simulink model "gaussian"  (R2017a)
settings: Solver=FixedStepDiscrete  StartTime=0.0  StopTime=10.0  RelTol=1e-3
undefined symbols (not defined in the file): gray, none, videoinput
libraries: imaqlib x1, visionfilter x1, visiontransforms x1, visiongeotforms x1, dspmtrx3 x1
settings Model: SimulationMode=accelerator  Creator=eruffaldi  LastModifiedBy=eruffaldi

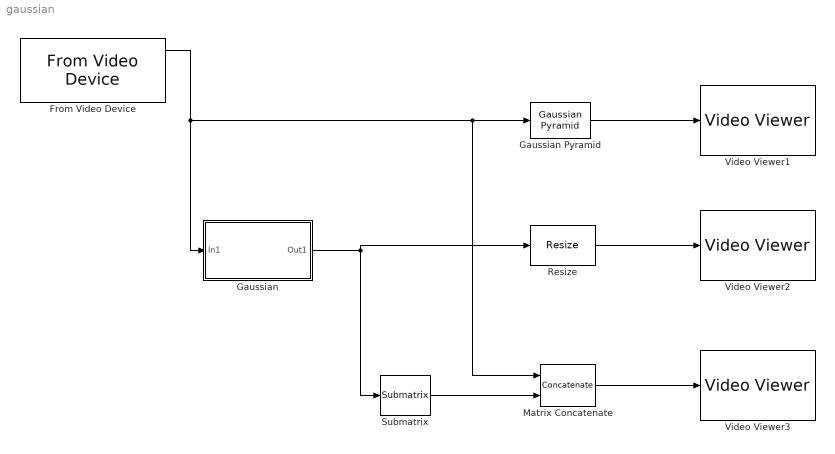
== system gaussian ==
  From Video Device : imaqlib/From Video Device  DeviceMenu=macvideo 1 (FaceTime HD Camera)  Device=macvideo 1 (FaceTime HD Camera)  ObjConstructor=videoinput('macvideo', 1)  VideoFormatMenu=YCbCr422_1280x720  VideoFormat=YCbCr422_1280x720  VideoSource=default  ROIPosition=[0 0 720 1280]  EnableHWTrigger=off  TriggerConfiguration=none/none  SampleTime=1/30  OutputPortsMode=Separate color signals  DataType=single  CanDoHWTrigger=no  ReturnedColorSpace=YCbCr  BlockHandle=2235.0077  ROIWidth=1280  ROIHeight=720  ROIColumn=0  ROIRow=0  EngXMLPath=/Applications/MATLAB_R2017a.app/toolbox/imaq/imaq/private  DevXMLPath=/Users/eruffaldi/Documents/MATLAB/SupportPackages/R2017a/toolbox/imaq/supportpackages/genericvideo/adaptor/maci64  EngLibPath=/Applications/MATLAB_R2017a.app/toolbox/imaq/imaqblks/imaqmex/maci64  ColorSpace=YCbCr  BayerSensorAlignment=grbg
      settings: SourceProductName=Image Acquisition Toolbox
  "Gaussian " : Subsystem
  Gaussian Pyramid : visiontransforms/Gaussian Pyramid  operation=Reduce  level=1  source="Default separable filter [1/4-a/2  1/4  a  1/4  1/4-a/2]"  a=0.375  coef=[0.0625 0.25 0.375 0.25 0.0625]  hiddenCoef=[1/4-0.375/2 1/4 0.375 1/4 1/4-0.375/2]  firstCoeffMode=Specify word length  firstCoeffWordLength=16  firstCoeffFracLength=16  outputMode=Binary point scaling  outputWordLength=32  outputFracLength=10  prodOutputMode=Binary point scaling  prodOutputWordLength=32  prodOutputFracLength=10  roundingMode=Floor  overflowMode=off
      settings: SourceProductName=Computer Vision System Toolbox  SourceProductBaseCode=VP
  Matrix Concatenate : Concatenate  Mode=Multidimensional array  ConcatenateDimension=2
  Resize : visiongeotforms/Resize  specify=Output size as a percentage of input size  rfactor=[50 50]  outCols=25  outRows=25  outRowsCols=[25 35]  interp_method=Nearest neighbor  antialias=on  useROI=off  roiFlag=off  prodOutputMode=Binary point scaling  prodOutputWordLength=32  prodOutputFracLength=10  roundingMode=Nearest  overflowMode=on
      settings: SourceProductName=Computer Vision System Toolbox  SourceProductBaseCode=VP
  Submatrix : dspmtrx3/Submatrix  RowSpan=Range of rows  RowStartMode=Index  RowStartIndex=3  RowEndMode=Offset from last  RowEndIndex=2  ColSpan=Range of columns  ColStartMode=Index  ColStartIndex=3  ColEndMode=Offset from last  ColEndIndex=2
  Video Viewer1 : VideoViewer  colormapValue=gray(256)  FigPos=[1503 788 846 595]
  Video Viewer2 : VideoViewer  colormapValue=gray(256)  FigPos=[2269 1000 846 595]
  Video Viewer3 : VideoViewer  colormapValue=gray(256)  FigPos=[1657 1046 1181 764]
  wires:
  From Video Device/1 -> "Gaussian "/1(In1), Matrix Concatenate/1, Gaussian Pyramid/1
  Resize/1 -> Video Viewer2/1
  Gaussian Pyramid/1 -> Video Viewer1/1
  Matrix Concatenate/1 -> Video Viewer3/1
  Submatrix/1 -> Matrix Concatenate/2
  "Gaussian "/1(Out1) -> Resize/1, Submatrix/1

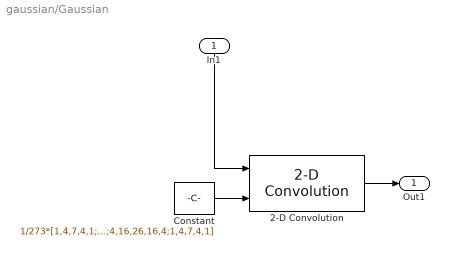
== system gaussian/Gaussian  ==
  In1 : Inport
  2-D Convolution : visionfilter/2-D Convolution  outSize=Full  normalize=off  outputMode=Binary point scaling  outputWordLength=32  outputFracLength=12  prodOutputMode=Binary point scaling  prodOutputWordLength=32  prodOutputFracLength=10  roundingMode=Floor  overflowMode=off
      settings: SourceProductName=Computer Vision System Toolbox  SourceProductBaseCode=VP
  Constant : Constant  Value=1/273*[1,4,7,4,1;4,16,26,16,4;7,26,41,26,7;4,16,26,16,4;1,4,7,4,1]  OutDataTypeStr=single
  Out1 : Outport
  wires:
  In1/1 -> 2-D Convolution/1
  2-D Convolution/1 -> Out1/1
  Constant/1 -> 2-D Convolution/2
